simulink model "model"  (R2025a)
settings: Solver=ode4  StartTime=0.0  StopTime=3500  FixedStep=0.01  RelTol=1e-3
values from neighbouring files (symbols this model uses):
  b = 1    [params.m]
  gmst0_deg = mod(gmst0_deg, 360.0)    [ic.m]
  J = [1 0 0 ... (first row only)    [params.m]
  JD_UTC = floor(365.25 * (Y + 4716))         + floor(30.6001 * (Mo + 1))         + D + B - 1524.5         + (h + mi/60 + s/3600) / 24    [ic.m]
  Jw = 1    [params.m]
  Kd = 2 * omega_n * zeta * J    [params.m]
  Ke = 1    [params.m]
  Kp = 2 * omega_n^2 * J    [params.m]
  Kt = 1    [params.m]
  L = 1    [params.m]
  q0 = q0 / norm(q0)    [ic.m]    (also in test.m = (C_B_ECI(1,2) - C_B_ECI(2,1)) * k)
  R = 1    [params.m]
  r0_I = orbit.ic.r0_I    [ic.m]
  trgt_ecef = [(N+h)*cos(lat)*cos(lon) ... (first row only)    [constants.m]    (also in test.m = trgt_ecef(:))
  v0_I = orbit.ic.v0_I    [ic.m]
  w0 = [0; 0; 0]    [ic.m]
undefined symbols (not defined in the file or in its folder): earth, weight_B, weight_S, WMM2025
libraries: vrlib x13, aerolibutil x3, simulink_extras x2, simulink x1, aerolibatmos2 x1, aerolibgravity2 x1
settings Model: Creator=procyon  LastModifiedBy=procyon

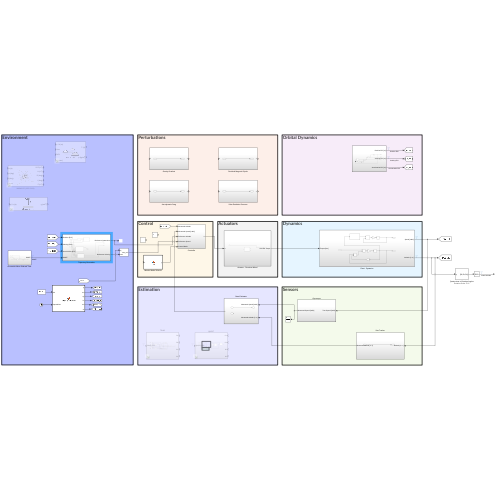
[thumbnail: Simulink's stored preview of the top-level diagram]
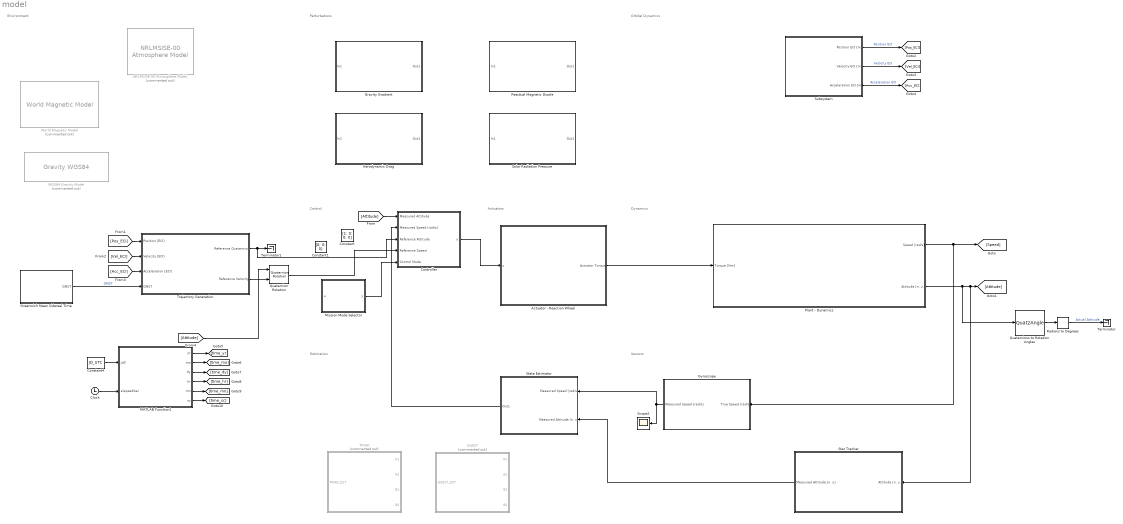
== system model ==
  note: Orbital Dynamics
  note: Environment
  note: Estimation
  note: Sensors
  note: Perturbations
  note: Control
  note: Actuators
  note: Dynamics
  Actuator - Reaction Wheel : Subsystem
  Aerodynamic Drag : Subsystem
  Clock : Clock
  Constant : Constant  Value=[1; 0; 0; 0]
  Constant1 : Constant  Value=[0; 0; 0]
  Constant4 : Constant  Value=JD_UTC
  Controller : Subsystem
  Gravity Gradient : Subsystem
  Greenwich Mean Sidereal Time : Subsystem
  Gyroscope : Subsystem
  MATLAB Function1 : MATLAB Function  TreatAsAtomicUnit=on
  Mission Mode Selector : MATLAB Function  TreatAsAtomicUnit=on
  NRLMSISE-00 Atmosphere Model : aerolibatmos2/NRLMSISE-00 Atmosphere Model  Commented=on  units=Metric (MKS)  lst_input=off  flux_ap_input=off  flags_input=Internal  flags=ones(1,23)  oxygen_in=off  action=Warning
  Plant - Dynamics : Subsystem
  QUEST : Subsystem  Commented=on
  Quaternion Rotation : aerolibutil/Quaternion Rotation
  Quaternions to Rotation Angles : Quat2Angle
      settings: AttributesFormatString=Rotation Order: %<rotationOrder>
  Radians to Degrees : simulink_extras/Transformations/Radians to Degrees
  Residual Magnetic Dipole : Subsystem
  Scope2 : Scope
      settings: ActiveDisplayYMinimum=-0.011319959817313957  ActiveDisplayYMaximum=0.0053397465657156794  DataLoggingVariableName=ScopeData2
  Solar Radiation Pressure : Subsystem
  Star Tracker : Subsystem
  State Estimator : Subsystem
  Subsystem : Subsystem
  TRIAD : Subsystem  Commented=on
  Terminator : Terminator
  Terminator1 : Terminator
  Trajectory Generation : Subsystem
  "WGS84 Gravity Model  " : GravityWGS84  Commented=on
  World Magnetic Model : aerolibgravity2/World Magnetic Model  Commented=on  model=WMM2025 (2025-2030)  customFile='WMM2025.COF'  units=Metric (MKS)  time_in=on  month=January  day=1  year=2025  action=Error  h_out=on  dec_out=on  inc_out=on  ti_out=on
  wires:
  Plant - Dynamics/1(Speed [rad/s]) -> [Speed], Gyroscope/1(True Speed [rad/s])
  Gyroscope/1(Measured Speed [rad/s]) -> State Estimator/1(Measured Speed [rad/s]), Scope2/1
  Mission Mode Selector/1(y) -> Controller/5(Control Mode)
  Actuator - Reaction Wheel/1(Actuator Torque) -> Plant - Dynamics/1(Torque [Nm])
  Controller/1(u) -> Actuator - Reaction Wheel/1(u)
  Plant - Dynamics/2(Attitude [n. u.]) -> Quaternions to Rotation Angles/1, Star Tracker/1(Attitude [n. u.]), [Attitude]
  [Attitude] -> Controller/1(Measured Attitude)
  Quaternions to Rotation Angles/1 -> Radians to Degrees/1
  Radians to Degrees/1 -> Terminator/1  "Actual Attitude"
  State Estimator/1(Out1) -> Controller/2(Measured Speed [rad/s])
  Star Tracker/1(Measured Attitude [n. u]) -> State Estimator/2(Measured Attitude [n. u])
  Subsystem/1(Position ECI [m]) -> [Pos_ECI]  "Position ECI"
  Subsystem/3(Acceleration ECI [m]) -> [Acc_ECI]  "Acceleration ECI"
  Subsystem/2(Velocity ECI [m]) -> [Vel_ECI]  "Velocity ECI"
  Greenwich Mean Sidereal Time/1(GMST) -> Trajectory Generation/4(GMST)  "GMST"
  MATLAB Function1/1(yr) -> [time_yr]
  MATLAB Function1/2(mo) -> [time_mo]
  MATLAB Function1/3(dy) -> [time_dy]
  MATLAB Function1/4(hr) -> [time_hr]
  MATLAB Function1/5(mn) -> [time_mn]
  MATLAB Function1/6(sc) -> [time_sc]
  Constant4/1 -> MATLAB Function1/1(jd0)
  Clock/1 -> MATLAB Function1/2(elapsedSec)
  [Pos_ECI] -> Trajectory Generation/1(Position [ECI])
  [Vel_ECI] -> Trajectory Generation/2(Velocity [ECI])
  [Acc_ECI] -> Trajectory Generation/3(Acceleration [ECI])
  Trajectory Generation/1(Reference Quaternion) -> Controller/3(Reference Attitude), Terminator1/1
  Trajectory Generation/2(Reference Velocity) -> Quaternion Rotation/2
  [Attitude] -> Quaternion Rotation/1
  Quaternion Rotation/1 -> Controller/4(Reference Speed)

== system model/Actuator - Reaction Wheel ==
  u : Inport
  DC Motor : Subsystem
  Actuator Torque : Outport
  wires:
  u/1 -> Actuator Torque/1

== system model/Aerodynamic Drag ==
  In1 : Inport
  Out1 : Outport
  wires:
  In1/1 -> Out1/1

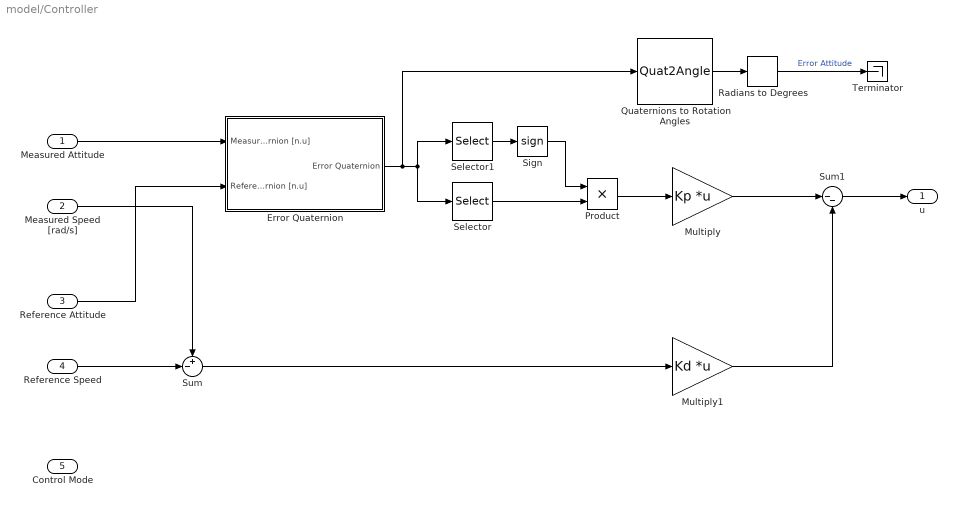
== system model/Controller ==
  Measured Attitude : Inport
  Measured Speed [rad/s] : Inport  Port=2
  Reference Attitude : Inport  Port=3
  Reference Speed : Inport  Port=4
  Control Mode : Inport  Port=5
  Error Quaternion : Subsystem
  Multiply : Gain  Gain=Kp  Multiplication=Matrix(K*u) (u vector)
  Multiply1 : Gain  Gain=Kd  Multiplication=Matrix(K*u) (u vector)
  Product : Product
  Quaternions to Rotation Angles : Quat2Angle
      settings: AttributesFormatString=Rotation Order: %<rotationOrder>
  Radians to Degrees : simulink_extras/Transformations/Radians to Degrees
  Selector : Selector  InputPortWidth=4  IndexOptions=Index vector (dialog)  Indices=[2 3 4]  OutputSizes=1
  Selector1 : Selector  InputPortWidth=4  IndexOptions=Index vector (dialog)  Indices=[1]  OutputSizes=1
  Sign : Signum
  Sum : Sum  Inputs=+-|
  Sum1 : Sum  Inputs=|--
  Terminator : Terminator
  u : Outport
  wires:
  Measured Attitude/1 -> Error Quaternion/1(Measured Quaternion [n.u])
  Reference Attitude/1 -> Error Quaternion/2(Reference Quaternion [n.u])
  Measured Speed [rad/s]/1 -> Sum/1
  Reference Speed/1 -> Sum/2
  Selector1/1 -> Sign/1
  Selector/1 -> Product/2
  Sign/1 -> Product/1
  Product/1 -> Multiply/1
  Sum/1 -> Multiply1/1
  Multiply/1 -> Sum1/1
  Multiply1/1 -> Sum1/2
  Sum1/1 -> u/1
  Quaternions to Rotation Angles/1 -> Radians to Degrees/1
  Radians to Degrees/1 -> Terminator/1  "Error Attitude"
  Error Quaternion/1(Error Quaternion) -> Quaternions to Rotation Angles/1, Selector1/1, Selector/1

== system model/Gravity Gradient ==
  In1 : Inport
  Out1 : Outport
  wires:
  In1/1 -> Out1/1

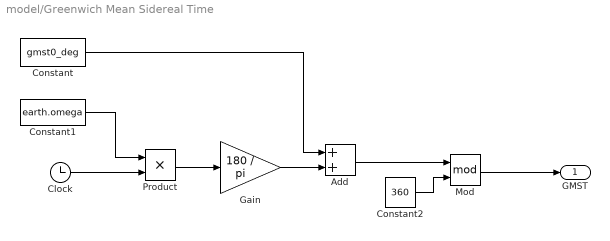
== system model/Greenwich Mean Sidereal Time ==
  Add : Sum
  Clock : Clock
  Constant : Constant  Value=gmst0_deg
  Constant1 : Constant  Value=earth.omega
  Constant2 : Constant  Value=360
  Gain : Gain  Gain=180 / pi
  Mod : Math  Operator=mod
  Product : Product
  GMST : Outport
  wires:
  Clock/1 -> Product/2
  Constant1/1 -> Product/1
  Product/1 -> Gain/1
  Gain/1 -> Add/2
  Constant/1 -> Add/1
  Mod/1 -> GMST/1
  Add/1 -> Mod/1
  Constant2/1 -> Mod/2

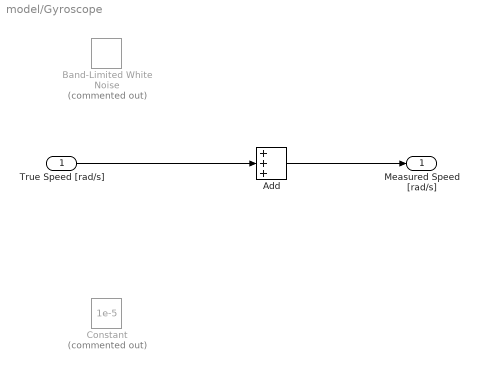
== system model/Gyroscope ==
  True Speed [rad/s] : Inport
  Add : Sum  Inputs=+++
  Band-Limited White Noise : simulink/Sources/Band-Limited White Noise  Commented=on  Cov=5e-8  Ts=0.01  seed=[23341]
  Constant : Constant  Commented=on  Value=1e-5
  Measured Speed [rad/s] : Outport
  wires:
  True Speed [rad/s]/1 -> Add/2
  Add/1 -> Measured Speed [rad/s]/1

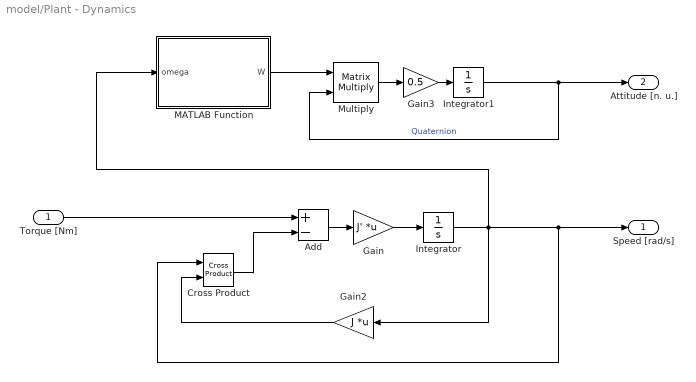
== system model/Plant - Dynamics ==
  Torque [Nm] : Inport
  Add : Sum  Inputs=+-
  Cross Product : vrlib/Utilities/Cross Product
  Gain : Gain  Gain=J'  Multiplication=Matrix(K*u)
  Gain2 : Gain  Gain=J  Multiplication=Matrix(K*u)
  Gain3 : Gain  Gain=0.5
  Integrator : Integrator  InitialCondition=w0
  Integrator1 : Integrator  InitialCondition=q0
  MATLAB Function : MATLAB Function  TreatAsAtomicUnit=on
  Multiply : Product  Inputs=**  Multiplication=Matrix(*)
  Speed [rad/s] : Outport
  Attitude [n. u.] : Outport  Port=2
  wires:
  Add/1 -> Gain/1
  Cross Product/1 -> Add/2
  Gain2/1 -> Cross Product/2
  Integrator/1 -> MATLAB Function/1(omega), Cross Product/1, Speed [rad/s]/1, Gain2/1
  MATLAB Function/1(W) -> Multiply/1
  Multiply/1 -> Gain3/1
  Integrator1/1 -> Attitude [n. u.]/1, Multiply/2  "Quaternion"
  Gain3/1 -> Integrator1/1
  Gain/1 -> Integrator/1
  Torque [Nm]/1 -> Add/1

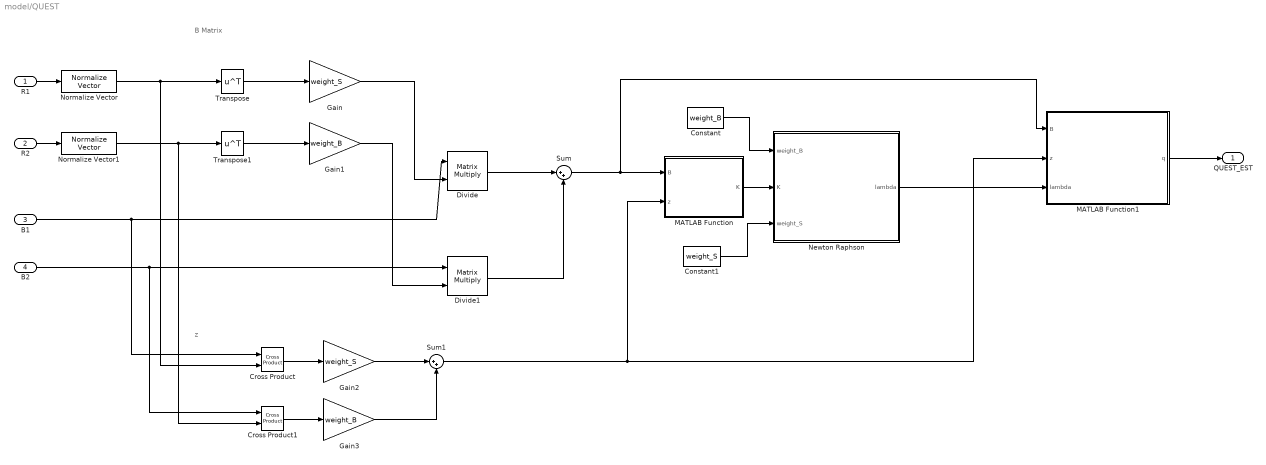
== system model/QUEST ==
  note: z
  note: B Matrix
  R1 : Inport
  R2 : Inport  Port=2
  B1 : Inport  Port=3
  B2 : Inport  Port=4
  Constant : Constant  Value=weight_B
  Constant1 : Constant  Value=weight_S
  Cross Product : vrlib/Utilities/Cross Product
  Cross Product1 : vrlib/Utilities/Cross Product
  Divide : Product  Inputs=**  Multiplication=Matrix(*)
  Divide1 : Product  Inputs=**  Multiplication=Matrix(*)
  Gain : Gain  Gain=weight_S
  Gain1 : Gain  Gain=weight_B
  Gain2 : Gain  Gain=weight_S
  Gain3 : Gain  Gain=weight_B
  MATLAB Function : MATLAB Function  TreatAsAtomicUnit=on
  MATLAB Function1 : MATLAB Function  TreatAsAtomicUnit=on
  Newton Raphson : MATLAB Function  TreatAsAtomicUnit=on
  Normalize Vector : vrlib/Utilities/Normalize Vector  maxzero=0
  Normalize Vector1 : vrlib/Utilities/Normalize Vector  maxzero=0
  Sum : Sum  Inputs=|++
  Sum1 : Sum  Inputs=|++
  Transpose : Math  Operator=transpose
  Transpose1 : Math  Operator=transpose
  QUEST_EST : Outport
  wires:
  R1/1 -> Normalize Vector/1
  R2/1 -> Normalize Vector1/1
  Normalize Vector/1 -> Cross Product/2, Transpose/1
  Transpose/1 -> Gain/1
  Transpose1/1 -> Gain1/1
  Divide/1 -> Sum/1
  Divide1/1 -> Sum/2
  Gain1/1 -> Divide1/2
  Gain/1 -> Divide/2
  B1/1 -> Cross Product/1, Divide/1
  Cross Product/1 -> Gain2/1
  Normalize Vector1/1 -> Cross Product1/2, Transpose1/1
  Cross Product1/1 -> Gain3/1
  B2/1 -> Cross Product1/1, Divide1/1
  Gain2/1 -> Sum1/1
  Gain3/1 -> Sum1/2
  Sum/1 -> MATLAB Function/1(B), MATLAB Function1/1(B)
  Sum1/1 -> MATLAB Function1/2(z), MATLAB Function/2(z)
  MATLAB Function/1(K) -> Newton Raphson/2(K)
  Constant/1 -> Newton Raphson/1(weight_B)
  Constant1/1 -> Newton Raphson/3(weight_S)
  Newton Raphson/1(lambda) -> MATLAB Function1/3(lambda)
  MATLAB Function1/1(q) -> QUEST_EST/1

== system model/Residual Magnetic Dipole ==
  In1 : Inport
  Out1 : Outport
  wires:
  In1/1 -> Out1/1

== system model/Solar Radiation Pressure ==
  In1 : Inport
  Out1 : Outport
  wires:
  In1/1 -> Out1/1

== system model/Star Tracker ==
  Attitude [n. u.] : Inport
  Measured Attitude [n. u] : Outport
  wires:
  Attitude [n. u.]/1 -> Measured Attitude [n. u]/1

== system model/State Estimator ==
  Measured Speed [rad/s] : Inport
  Measured Attitude [n. u] : Inport  Port=2
  Out1 : Outport
  wires:
  Measured Speed [rad/s]/1 -> Out1/1

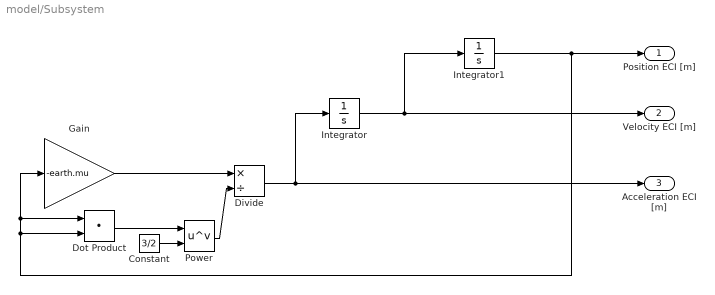
== system model/Subsystem ==
  Constant : Constant  Value=3/2
  Divide : Product  Inputs=*/
  Dot Product : DotProduct  OutDataTypeStr=Inherit: Inherit via internal rule
  Gain : Gain  Gain=-earth.mu
  Integrator : Integrator  InitialCondition=v0_I
  Integrator1 : Integrator  InitialCondition=r0_I
  Power : Math  Operator=pow
  Position ECI [m] : Outport
  Velocity ECI [m] : Outport  Port=2
  Acceleration ECI [m] : Outport  Port=3
  wires:
  Integrator/1 -> Integrator1/1, Velocity ECI [m]/1
  Integrator1/1 -> Dot Product/2, Dot Product/1, Gain/1, Position ECI [m]/1
  Dot Product/1 -> Power/1
  Gain/1 -> Divide/1
  Divide/1 -> Integrator/1, Acceleration ECI [m]/1
  Constant/1 -> Power/2
  Power/1 -> Divide/2

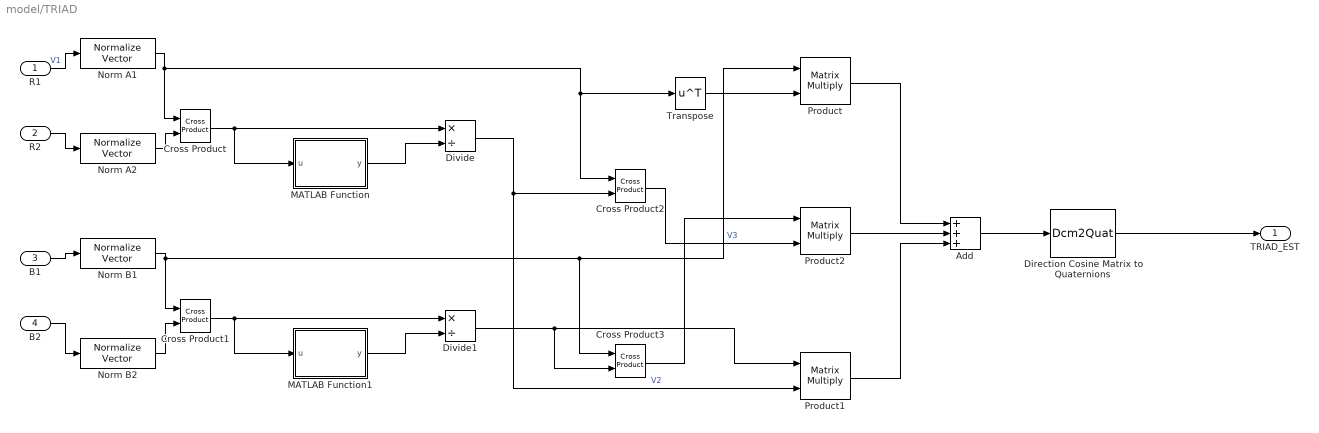
== system model/TRIAD ==
  R1 : Inport
  R2 : Inport  Port=2
  B1 : Inport  Port=3
  B2 : Inport  Port=4
  Add : Sum  Inputs=+++
  Cross Product{,1..3} (4 alike) : vrlib/Utilities/Cross Product
  Direction Cosine Matrix to Quaternions : Dcm2Quat  action=Warning
  Divide : Product  Inputs=*/
  Divide1 : Product  Inputs=*/
  MATLAB Function : MATLAB Function  TreatAsAtomicUnit=on
  MATLAB Function1 : MATLAB Function  TreatAsAtomicUnit=on
  Norm A1 : vrlib/Utilities/Normalize Vector  maxzero=0
  Norm A2 : vrlib/Utilities/Normalize Vector  maxzero=0
  Norm B1 : vrlib/Utilities/Normalize Vector  maxzero=0
  Norm B2 : vrlib/Utilities/Normalize Vector  maxzero=0
  Product : Product  Multiplication=Matrix(*)
  Product1 : Product  Multiplication=Matrix(*)
  Product2 : Product  Multiplication=Matrix(*)
  Transpose : Math  Operator=transpose
  TRIAD_EST : Outport
  wires:
  Direction Cosine Matrix to Quaternions/1 -> TRIAD_EST/1
  R1/1 -> Norm A1/1  "V1"
  R2/1 -> Norm A2/1
  Cross Product/1 -> MATLAB Function/1(u), Divide/1
  MATLAB Function/1(y) -> Divide/2
  Cross Product1/1 -> MATLAB Function1/1(u), Divide1/1
  B1/1 -> Norm B1/1
  MATLAB Function1/1(y) -> Divide1/2
  B2/1 -> Norm B2/1
  Divide/1 -> Product1/2, Cross Product2/2  "V2"
  Divide1/1 -> Product1/1, Cross Product3/2
  Transpose/1 -> Product/2
  Cross Product3/1 -> Product2/1
  Cross Product2/1 -> Product2/2  "V3"
  Product2/1 -> Add/2
  Product/1 -> Add/1
  Product1/1 -> Add/3
  Add/1 -> Direction Cosine Matrix to Quaternions/1
  Norm A2/1 -> Cross Product/2
  Norm B2/1 -> Cross Product1/2
  Norm A1/1 -> Transpose/1, Cross Product2/1, Cross Product/1
  Norm B1/1 -> Product/1, Cross Product3/1, Cross Product1/1

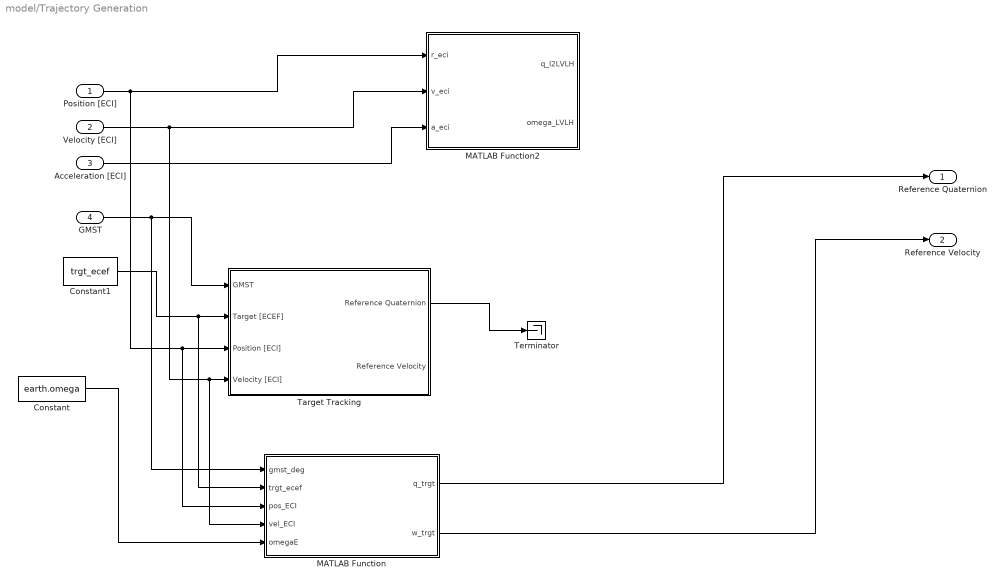
== system model/Trajectory Generation ==
  Position [ECI] : Inport
  Velocity [ECI] : Inport  Port=2
  Acceleration [ECI] : Inport  Port=3
  GMST : Inport  Port=4
  Constant : Constant  Value=earth.omega
  Constant1 : Constant  Value=trgt_ecef
  MATLAB Function : MATLAB Function  TreatAsAtomicUnit=on
  MATLAB Function2 : MATLAB Function  TreatAsAtomicUnit=on
  Target Tracking : Subsystem
  Terminator : Terminator
  Reference Quaternion : Outport
  Reference Velocity : Outport  Port=2
  wires:
  Position [ECI]/1 -> MATLAB Function/3(pos_ECI), Target Tracking/3(Position [ECI]), MATLAB Function2/1(r_eci)
  Velocity [ECI]/1 -> MATLAB Function/4(vel_ECI), Target Tracking/4(Velocity [ECI]), MATLAB Function2/2(v_eci)
  Acceleration [ECI]/1 -> MATLAB Function2/3(a_eci)
  Target Tracking/1(Reference Quaternion) -> Terminator/1
  Constant1/1 -> MATLAB Function/2(trgt_ecef), Target Tracking/2(Target [ECEF])
  GMST/1 -> MATLAB Function/1(gmst_deg), Target Tracking/1(GMST)
  Constant/1 -> MATLAB Function/5(omegaE)
  MATLAB Function/1(q_trgt) -> Reference Quaternion/1
  MATLAB Function/2(w_trgt) -> Reference Velocity/1

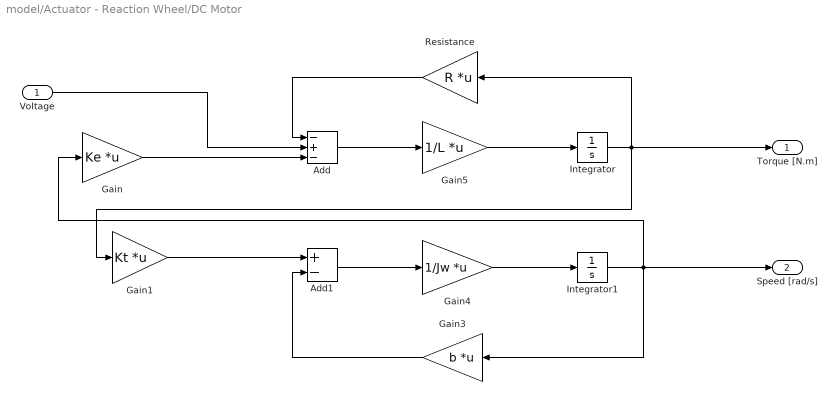
== system model/Actuator - Reaction Wheel/DC Motor ==
  Voltage : Inport
  Add : Sum  Inputs=-+-
  Add1 : Sum  Inputs=+-
  Gain : Gain  Gain=Ke  Multiplication=Matrix(K*u) (u vector)
  Gain1 : Gain  Gain=Kt  Multiplication=Matrix(K*u) (u vector)
  Gain3 : Gain  Gain=b  Multiplication=Matrix(K*u) (u vector)
  Gain4 : Gain  Gain=1/Jw  Multiplication=Matrix(K*u) (u vector)
  Gain5 : Gain  Gain=1/L  Multiplication=Matrix(K*u) (u vector)
  Integrator : Integrator
  Integrator1 : Integrator
  Resistance : Gain  Gain=R  Multiplication=Matrix(K*u) (u vector)
  Torque [N.m] : Outport
  Speed [rad/s] : Outport  Port=2
  wires:
  Voltage/1 -> Add/2
  Gain/1 -> Add/3
  Resistance/1 -> Add/1
  Gain1/1 -> Add1/1
  Gain3/1 -> Add1/2
  Add1/1 -> Gain4/1
  Add/1 -> Gain5/1
  Gain5/1 -> Integrator/1
  Gain4/1 -> Integrator1/1
  Integrator/1 -> Torque [N.m]/1, Gain1/1, Resistance/1
  Integrator1/1 -> Gain/1, Speed [rad/s]/1, Gain3/1

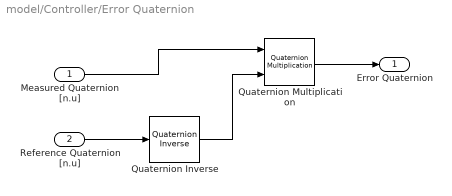
== system model/Controller/Error Quaternion ==
  Measured Quaternion [n.u] : Inport
  Reference Quaternion [n.u] : Inport  Port=2
  Quaternion Inverse : aerolibutil/Quaternion Inverse
  Quaternion Multiplication : aerolibutil/Quaternion Multiplication
  Error Quaternion : Outport
  wires:
  Reference Quaternion [n.u]/1 -> Quaternion Inverse/1
  Quaternion Multiplication/1 -> Error Quaternion/1
  Quaternion Inverse/1 -> Quaternion Multiplication/2
  Measured Quaternion [n.u]/1 -> Quaternion Multiplication/1

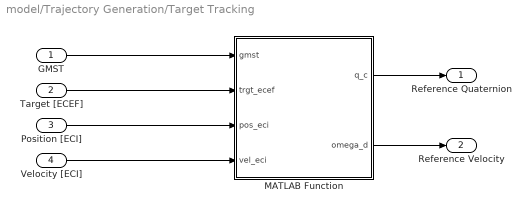
== system model/Trajectory Generation/Target Tracking ==
  GMST : Inport
  Target [ECEF] : Inport  Port=2
  Position [ECI] : Inport  Port=3
  Velocity [ECI] : Inport  Port=4
  MATLAB Function : MATLAB Function  TreatAsAtomicUnit=on
  Reference Quaternion : Outport
  Reference Velocity : Outport  Port=2
  wires:
  GMST/1 -> MATLAB Function/1(gmst)
  Target [ECEF]/1 -> MATLAB Function/2(trgt_ecef)
  Position [ECI]/1 -> MATLAB Function/3(pos_eci)
  MATLAB Function/1(q_c) -> Reference Quaternion/1
  MATLAB Function/2(omega_d) -> Reference Velocity/1
  Velocity [ECI]/1 -> MATLAB Function/4(vel_eci)

== matlab function model/QUEST/MATLAB Function1 ==
  data: B input; q output; z input; lambda input
function q = quest_qopt(B, z, lambda)
% q_opt from B, z, lambda where rho = lambda + tr(B)
% q = [q1;q2;q3;q4] (normalized; flips sign to make q4 >= 0)

    % checks
    if ~isequal(size(B),[3 3]); error('B must be 3x3'); end
    z = z(:);
    if ~isequal(size(z),[3 1]); error('z must be 3x1'); end

    trB = trace(B);
    S   = B + B.';
    rho = lambda + trB;
    A   = rho*eye(3) - S;

    % adj(A) via cofactors (works even if A is singular)
    a=A(1,1); b=A(1,2); c=A(1,3);
    d=A(2,1); e=A(2,2); f=A(2,3);
    g=A(3,1); h=A(3,2); i=A(3,3);
    adjA = [ e*i - f*h,  c*h - b*i,  b*f - c*e;
             f*g - d*i,  a*i - c*g,  c*d - a*f;
             d*h - e*g,  b*g - a*h,  a*e - b*d ];

    top  = adjA * z;
    bot  = det(A);

    q = [top; bot];
    n = norm(q);
    if ~isfinite(n) || n == 0
        error('Degenerate inputs');
    end
    q = q / n;
    if q(4) < 0, q = -q; end

    q = [q(4); q(1:3)];
    
end

== matlab function model/Mission Mode Selector ==
  data: u input; y output
function y = fcn(u)

y = u;

== matlab function model/Plant - Dynamics/MATLAB Function ==
  data: omega input; W output
function W = omegaMat(omega)
%OMEGAMAT  Quaternion kinematic matrix (scalar-first convention)
%
%   W = omegaMat(omega)
%
% Builds the 4x4 matrix W(omega) such that:
%       q_dot = 0.5 * W(omega) * q
%
% Inputs:
%   omega : 3x1 angular velocity vector [rad/s] in body frame
%
% Output:
%   W     : 4x4 quaternion kinematic matrix (scalar-first convention)
%
%   Using the definition:
%       W(ω) = [  0      -ωᵀ
%                 ω   [ω×] ]

    % ensure column vector
    omega = omega(:);

    % skew-symmetric cross-product matrix
    omega_cross = [  0       -omega(3)   omega(2);
                  omega(3)     0        -omega(1);
                 -omega(2)   omega(1)     0      ];

    % assemble full 4x4 matrix
    W = [ 0          -omega.';
          omega       omega_cross ];
end

== matlab function model/Trajectory Generation/MATLAB Function2 ==
  data: r_eci input; q_I2LVLH output; v_eci input; a_eci input; omega_LVLH output
function [q_I2LVLH, omega_LVLH] = nadir_pointing(r_eci, v_eci, a_eci)
%#codegen
% Computes desired attitude quaternion and angular velocity for nadir pointing.
%
% Inputs:
%   r_eci  [3x1] - Position in ECI (m or km)
%   v_eci  [3x1] - Velocity in ECI
%   a_eci  [3x1] - Acceleration in ECI (including perturbations)
%
% Outputs:
%   q_I2LVLH    [4x1] - Desired quaternion (ECI -> Body=LVLH), scalar-first [q0 q1 q2 q3]
%   omega_LVLH  [3x1] - Desired angular velocity in LVLH frame (rad/s)

    %% Build LVLH basis vectors in ECI
    r_eci = r_eci(:);
    v_eci = v_eci(:);
    a_eci = a_eci(:);

    r_norm = norm(r_eci);
    h_vec  = cross(r_eci, v_eci);
    h_norm = norm(h_vec);

    % Nadir: +z_body = -r_hat (pointing toward Earth)
    e3 = -r_eci / r_norm;

    % -orbit normal
    e2 = -h_vec / h_norm;

    % Completes right-handed frame (~ velocity direction)
    e1 = cross(e2, e3);

    %% DCM: ECI -> LVLH (rows are the basis vectors)
    C = [e1'; e2'; e3'];

    %% Quaternion from DCM (Shepperd's method)
    q_I2LVLH = dcm2quat(C);

    %% Angular velocity via Cdot * C'
    % Time derivatives of the underlying vectors
    % d/dt(r) = v,  d/dt(r x v) = r x a

    % Derivative of e3 = -r_hat
    r_dot = v_eci;
    de3 = -(r_dot - e3 * dot(e3, r_dot)) / r_norm;

    % Derivative of e2 = -h_hat
    h_dot = cross(r_eci, a_eci);
    de2 = -(h_dot - e2 * dot(e2, h_dot)) / h_norm;

    % Derivative of e1 = e2 x e3
    de1 = cross(de2, e3) + cross(e2, de3);

    %% Skew-symmetric matrix [omega x] = Cdot * C^T
    Cdot = [de1'; de2'; de3'];
    S = Cdot * C';

    %% Extract angular velocity components (in LVLH frame)
    omega_LVLH = [S(3,2); S(1,3); S(2,1)];

end

%% ---- Helper: DCM to quaternion (Shepperd's method) ----
function q = dcm2quat(C)
    tr = C(1,1) + C(2,2) + C(3,3);

    q0 = 0.0;
    q1 = 0.0;
    q2 = 0.0;
    q3 = 0.0;

    vals = [tr, C(1,1), C(2,2), C(3,3)];
    [~, idx] = max(vals);

    switch idx
        case 1
            q0 = 0.5 * sqrt(1 + tr);
            k = 0.25 / q0;
            q1 = (C(2,3) - C(3,2)) * k;
            q2 = (C(3,1) - C(1,3)) * k;
            q3 = (C(1,2) - C(2,1)) * k;
        case 2
            q1 = 0.5 * sqrt(1 + 2*C(1,1) - tr);
            k = 0.25 / q1;
            q0 = (C(2,3) - C(3,2)) * k;
            q2 = (C(1,2) + C(2,1)) * k;
            q3 = (C(3,1) + C(1,3)) * k;
        case 3
            q2 = 0.5 * sqrt(1 + 2*C(2,2) - tr);
            k = 0.25 / q2;
            q0 = (C(3,1) - C(1,3)) * k;
            q1 = (C(1,2) + C(2,1)) * k;
            q3 = (C(2,3) + C(3,2)) * k;
        case 4
            q3 = 0.5 * sqrt(1 + 2*C(3,3) - tr);
            k = 0.25 / q3;
            q0 = (C(1,2) - C(2,1)) * k;
            q1 = (C(3,1) + C(1,3)) * k;
            q2 = (C(2,3) + C(3,2)) * k;
    end

    q = [q0; q1; q2; q3];

    % Enforce positive scalar part for consistency
    if q(1) < 0
        q = -q;
    end
end

== matlab function model/MATLAB Function1 ==
  data: jd0 input; yr output; elapsedSec input; mo output; dy output; hr output; mn output; sc output
function [yr, mo, dy, hr, mn, sc] = julianToCalendar(jd0, elapsedSec)
%#codegen
% Converts initial Julian Date + elapsed seconds to calendar date/time.
%
% Inputs:
%   jd0        - Initial epoch as Julian Date (days)
%   elapsedSec - Elapsed simulation time (seconds)
%
% Outputs:
%   yr, mo, dy, hr, mn, sc - Current UTC date and time

    % Current Julian Date
    jd = jd0 + elapsedSec / 86400;

    % Algorithm based on Meeus, "Astronomical Algorithms"
    jd_plus = jd + 0.5;
    Z = floor(jd_plus);
    F = jd_plus - Z;

    if Z < 2299161
        A = Z;
    else
        alpha = floor((Z - 1867216.25) / 36524.25);
        A = Z + 1 + alpha - floor(alpha / 4);
    end

    B = A + 1524;
    C = floor((B - 122.1) / 365.25);
    D = floor(365.25 * C);
    E = floor((B - D) / 30.6001);

    day_frac = B - D - floor(30.6001 * E) + F;
    dy = floor(day_frac);

    if E < 14
        mo = E - 1;
    else
        mo = E - 13;
    end

    if mo > 2
        yr = C - 4716;
    else
        yr = C - 4715;
    end

    % Extract h/m/s from fractional day
    frac = day_frac - dy;
    hr = floor(frac * 24);
    mn = floor((frac * 24 - hr) * 60);
    sc = (frac * 86400) - hr * 3600 - mn * 60;
end

== matlab function model/Trajectory Generation/Target Tracking/MATLAB Function ==
  settings: updateMethod=DISCRETE  sampleTime=0.05
  data: gmst input; trgt_ecef input; q_c output; pos_eci input; vel_eci input; omega_d output
function [q_c, omega_d] = quatCmd(gmst, trgt_ecef, pos_eci, vel_eci)
    persistent q_c_prev;
    q_c_prev = [1; 0; 0; 0];

    % Earth rotation rate (rad/s)
    omega_E = 7.2921159e-5;
    w_E = [0; 0; omega_E];

    % Target direction in ECI
    trgt_eci = ecef2eci(gmst, trgt_ecef);
    x_sit = trgt_eci - pos_eci;
    u_sit = x_sit / norm(x_sit);

    % Payload mounting axis (constant in body frame)
    u_com = [0; 0; 1];
    u_com = u_com / norm(u_com);

    % Rotation angle via atan2
    cp = cross(u_sit, u_com);
    dp = dot(u_sit, u_com);
    delta = atan2(norm(cp), dp);

    % Euler axis
    if norm(cp) < 1e-12
        if dp > 0
            q_c = [1; 0; 0; 0];
        else
            if abs(u_sit(1)) < 0.9
                perp = cross(u_sit, [1;0;0]);
            else
                perp = cross(u_sit, [0;1;0]);
            end
            q_c = [0; perp/norm(perp)];
        end
        omega_d = [0; 0; 0];
        return;
    end

    e_c = cp / norm(cp);

    % Commanded quaternion [scalar; vector] 
    q_c = [cos(delta/2); e_c * sin(delta/2)];

    % Enforce sign continuity
    if ~isempty(q_c_prev)
        if dot(q_c, q_c_prev) < 0
            q_c = -q_c;
        end
    end
    q_c_prev = q_c;

    % --- Desired angular velocity ---
    % Target velocity in ECI (fixed on rotating Earth)
    x_dot_sit = cross(w_E, trgt_eci) - vel_eci;

    % omega_d in ECI
    omega_d_eci = cross(x_sit, x_dot_sit) / dot(x_sit, x_sit);

    % Rotate to body frame using q_c
    omega_d = quatRot(q_c, omega_d_eci);
end

function v_rot = quatRot(q, v)
    % Rotate vector v by quaternion q (scalar-first: [w; x; y; z])
    % v_rot = q * [0;v] * q'
    w = q(1); x = q(2); y = q(3); z = q(4);
    
    t = 2 * cross([x;y;z], v);
    v_rot = v + w*t + cross([x;y;z], t);
end

function trgt_eci = ecef2eci(gmst, trgt_ecef)
    c = cos(gmst);
    s = sin(gmst);
    A = [c -s 0;
         s  c 0;
         0  0 1];
    trgt_eci = A * trgt_ecef;
end

== matlab function model/Trajectory Generation/MATLAB Function ==
  data: gmst_deg input; q_trgt output; trgt_ecef input; pos_ECI input; vel_ECI input; omegaE input; w_trgt output
function [q_trgt, w_trgt] = quatCmd(gmst_deg, trgt_ecef, pos_ECI, vel_ECI, omegaE)

q_trgt = zeros(4,1);
w_trgt = zeros(3,1);
I3 = eye(3);

% -------- ECEF -> ECI (from GMST) --------
th = gmst_deg * (pi/180);
c  = cos(th);
s  = sin(th);

C_ECI_ECEF = [ c -s 0;
               s  c 0;
               0  0 1];

Cdot_ECI_ECEF = omegaE * [ -s -c 0;
                             c -s 0;
                             0  0 0 ];

trgt_ecef = trgt_ecef(:);
trgt_eci  = C_ECI_ECEF * trgt_ecef;

% -------- Inputs --------
r_ECI = pos_ECI(:);
v_ECI = vel_ECI(:);

if ~all(isfinite([r_ECI; v_ECI; trgt_ecef; gmst_deg; omegaE]))
    q_trgt = [1;0;0;0];
    w_trgt = [0;0;0];
    return;
end

% -------- LVLH axes --------
r_norm = norm(r_ECI);
h_ECI  = cross(r_ECI, v_ECI);
h_norm = norm(h_ECI);

if (r_norm <= eps) || (h_norm <= eps)
    q_trgt = [1;0;0;0];
    w_trgt = [0;0;0];
    return;
end

eR = -r_ECI / r_norm;
eW = -h_ECI / h_norm;
eS = cross(eW, eR);

nS = norm(eS);
if nS <= eps
    q_trgt = [1;0;0;0];
    w_trgt = [0;0;0];
    return;
end
eS = eS / nS;

eW = cross(eR, eS);
eW = eW / norm(eW);

C_LVLH_ECI = [eS.'; eW.'; eR.'];

% -------- LOS vector in LVLH --------
rho_ECI  = trgt_eci - r_ECI;
rho_norm = norm(rho_ECI);

if (~all(isfinite(rho_ECI))) || (rho_norm <= eps)
    q_trgt = [1;0;0;0];
    w_trgt = [0;0;0];
    return;
end

rho_LVLH = C_LVLH_ECI * rho_ECI;
rhoL_n   = norm(rho_LVLH);
if rhoL_n <= eps
    q_trgt = [1;0;0;0];
    w_trgt = [0;0;0];
    return;
end
u_los = rho_LVLH / rhoL_n;

% -------- Quaternion in LVLH: payload boresight -> LOS --------
u_payload = [0;0;1];
cdot = dot(u_payload, u_los);
cdot = min(1.0, max(-1.0, cdot));
delta = acos(cdot);

v_axis = cross(u_payload, u_los);
nva = norm(v_axis);
if nva < 1.0e-12
    if abs(u_los(3)) < 0.9
        tmp = [0;0;1];
    else
        tmp = [1;0;0];
    end
    v_axis = cross(u_payload, tmp);
    v_axis = v_axis / norm(v_axis);
else
    v_axis = v_axis / nva;
end

q_los_LVLH = [cos(0.5*delta);
              v_axis(1)*sin(0.5*delta);
              v_axis(2)*sin(0.5*delta);
              v_axis(3)*sin(0.5*delta)];
q_los_LVLH = q_los_LVLH / norm(q_los_LVLH);

% -------- Quaternion of LVLH wrt ECI from DCM --------
C = C_LVLH_ECI;
tr = C(1,1) + C(2,2) + C(3,3);
q_LVLH_ECI = zeros(4,1);

if tr > 0
    S = sqrt(max(tr + 1.0, 0)) * 2;
    q_LVLH_ECI(1) = 0.25 * S;
    q_LVLH_ECI(2) = (C(3,2) - C(2,3)) / S;
    q_LVLH_ECI(3) = (C(1,3) - C(3,1)) / S;
    q_LVLH_ECI(4) = (C(2,1) - C(1,2)) / S;
else
    if (C(1,1) > C(2,2)) && (C(1,1) > C(3,3))
        S = sqrt(max(1.0 + C(1,1) - C(2,2) - C(3,3), 0)) * 2;
        q_LVLH_ECI(1) = (C(3,2) - C(2,3)) / S;
        q_LVLH_ECI(2) = 0.25 * S;
        q_LVLH_ECI(3) = (C(1,2) + C(2,1)) / S;
        q_LVLH_ECI(4) = (C(1,3) + C(3,1)) / S;
    elseif (C(2,2) > C(3,3))
        S = sqrt(max(1.0 + C(2,2) - C(1,1) - C(3,3), 0)) * 2;
        q_LVLH_ECI(1) = (C(1,3) - C(3,1)) / S;
        q_LVLH_ECI(2) = (C(1,2) + C(2,1)) / S;
        q_LVLH_ECI(3) = 0.25 * S;
        q_LVLH_ECI(4) = (C(2,3) + C(3,2)) / S;
    else
        S = sqrt(max(1.0 + C(3,3) - C(1,1) - C(2,2), 0)) * 2;
        q_LVLH_ECI(1) = (C(2,1) - C(1,2)) / S;
        q_LVLH_ECI(2) = (C(1,3) + C(3,1)) / S;
        q_LVLH_ECI(3) = (C(2,3) + C(3,2)) / S;
        q_LVLH_ECI(4) = 0.25 * S;
    end
end

q_LVLH_ECI = q_LVLH_ECI / norm(q_LVLH_ECI);

% -------- Compose: q_trgt = q_los_LVLH ⊗ q_LVLH_ECI --------
w1 = q_los_LVLH(1); x1 = q_los_LVLH(2); y1 = q_los_LVLH(3); z1 = q_los_LVLH(4);
w2 = q_LVLH_ECI(1); x2 = q_LVLH_ECI(2); y2 = q_LVLH_ECI(3); z2 = q_LVLH_ECI(4);

q_trgt(1) = w1*w2 - x1*x2 - y1*y2 - z1*z2;
q_trgt(2) = w1*x2 + x1*w2 + y1*z2 - z1*y2;
q_trgt(3) = w1*y2 - x1*z2 + y1*w2 + z1*x2;
q_trgt(4) = w1*z2 + x1*y2 - y1*x2 + z1*w2;

q_trgt = q_trgt / norm(q_trgt);

% -------- Desired angular velocity (ECI, simple form) --------
rho_dot_ECI = Cdot_ECI_ECEF * trgt_ecef - v_ECI;
w_trgt = cross(rho_ECI, rho_dot_ECI) / dot(rho_ECI, rho_ECI);

end

== matlab function model/TRIAD/MATLAB Function ==
  data: u input; y output
function y = l2norm(u)
%#codegen
% Euclidean (L2) norm of a vector u
% Works for row or column vectors (double/single)

u = u(:);                  % force column
y = sqrt(sum(u .* u));     % ||u||_2 = sqrt(u'u)
end

== matlab function model/TRIAD/MATLAB Function1 ==
  data: u input; y output
function y = l2norm(u)
%#codegen
% Euclidean (L2) norm of a vector u
% Works for row or column vectors (double/single)

u = u(:);                  % force column
y = sqrt(sum(u .* u));     % ||u||_2 = sqrt(u'u)
end

== matlab function model/QUEST/Newton Raphson ==
  data: weight_B input; lambda output; K input; weight_S input
function lambda = fcn(weight_B, K, weight_S)
    % Newton–Raphson no polinômio característico de K
    coeffs     = poly(K);
    coeffs_der = polyder(coeffs);

    lambda = weight_B + weight_S;   % chute inicial
    max_iter  = 100;
    tol_f     = 1e-12;              % tolerância em f(lambda)
    tol_step  = 1e-12;              % tolerância no passo relativo

    for i = 1:max_iter
        f  = polyval(coeffs, lambda);
        fp = polyval(coeffs_der, lambda);

        if ~isfinite(fp) || fp == 0
            % Derivada zero/NaN: evite divisão por zero
            break
        end

        step   = f / fp;
        lambda_new = lambda - step;

        % Critérios de parada: valor da função e tamanho do passo
        if abs(f) < tol_f || abs(lambda_new - lambda) <= tol_step*(1+abs(lambda))
            lambda = lambda_new;
            break
        end

        lambda = lambda_new;
    end
end

== matlab function model/QUEST/MATLAB Function ==
  data: B input; K output; z input
function K = K_B(B, z)
% K(B) = [ B + B.' - (trace(B))*I3,  z ;
%          z.',                     trace(B) ]

    trB = trace(B);
    S   = B + B.';
    z   = z(:);              % ensure 3x1

    K = [ S - trB*eye(3), z ;
          z.',             trB ];
end
